simulink model "svpwm3level"  (Simulink 7.1)
settings: Solver=ode3  StartTime=0.0  StopTime=1  RelTol=1e-3
libraries: powerlib x13, simulink x1
(part 2 of 2)

== system svpwm3level/svpwm/Vector status/II/2-1 ==
  m : Inport  OutDataType=sfix(16)  OutScaling=2^0
  Constant1 : Constant  Value=[0 0 0]  OutDataType=sfix(16)  OutScaling=2^0
  Constant11 : Constant  Value=[0 0 0]  OutDataType=sfix(16)  OutScaling=2^0
  Constant12 : Constant  Value=[1 1 0]  OutDataType=sfix(16)  OutScaling=2^0
  Constant13 : Constant  Value=[0 1 0]  OutDataType=sfix(16)  OutScaling=2^0
  Constant2 : Constant  Value=[0 0 -1]  OutDataType=sfix(16)  OutScaling=2^0
  Constant3 : Constant  Value=[0 1 0]  OutDataType=sfix(16)  OutScaling=2^0
  Constant4 : Constant  Value=[1 1 0]  OutDataType=sfix(16)  OutScaling=2^0
  Multiport Switch : MultiPortSwitch  Inputs=7  OutDataType=sfix(16)  OutScaling=2^0  InputSameDT=on
  State : Outport  OutDataType=sfix(16)  OutScaling=2^0
  wires:
  Constant12/1 -> Multiport Switch/2
  Constant13/1 -> Multiport Switch/3
  Constant11/1 -> Multiport Switch/4
  m/1 -> Multiport Switch/1
  Multiport Switch/1 -> State/1
  Constant2/1 -> Multiport Switch/5
  Constant1/1 -> Multiport Switch/6
  Constant3/1 -> Multiport Switch/7
  Constant4/1 -> Multiport Switch/8

== system svpwm3level/svpwm/Vector status/II/2-2 ==
  m : Inport  OutDataType=sfix(16)  OutScaling=2^0
  Constant1 : Constant  Value=[0 0 -1]  OutDataType=sfix(16)  OutScaling=2^0
  Constant2 : Constant  Value=[0 0 0]  OutDataType=sfix(16)  OutScaling=2^0
  Constant3 : Constant  Value=[0 1 0]  OutDataType=sfix(16)  OutScaling=2^0
  Constant6 : Constant  Value=[0 0 -1]  OutDataType=sfix(16)  OutScaling=2^0
  Constant7 : Constant  Value=[0 1 0]  OutDataType=sfix(16)  OutScaling=2^0
  Constant8 : Constant  Value=[0 0 0]  OutDataType=sfix(16)  OutScaling=2^0
  Constant9 : Constant  Value=[-1 0 -1]  OutDataType=sfix(16)  OutScaling=2^0
  Multiport Switch1 : MultiPortSwitch  Inputs=7  OutDataType=sfix(16)  OutScaling=2^0  InputSameDT=on
  State1 : Outport  OutDataType=sfix(16)  OutScaling=2^0
  wires:
  Constant3/1 -> Multiport Switch1/8
  Constant2/1 -> Multiport Switch1/7
  Constant1/1 -> Multiport Switch1/6
  Constant9/1 -> Multiport Switch1/5
  Multiport Switch1/1 -> State1/1
  m/1 -> Multiport Switch1/1
  Constant6/1 -> Multiport Switch1/4
  Constant8/1 -> Multiport Switch1/3
  Constant7/1 -> Multiport Switch1/2

== system svpwm3level/svpwm/Vector status/II/2-3 ==
  m : Inport  OutDataType=sfix(16)  OutScaling=2^0
  Constant1 : Constant  Value=[1 1 0]  OutDataType=sfix(16)  OutScaling=2^0
  Constant11 : Constant  Value=[1 1 0]  OutDataType=sfix(16)  OutScaling=2^0
  Constant12 : Constant  Value=[1 1 -1]  OutDataType=sfix(16)  OutScaling=2^0
  Constant13 : Constant  Value=[0 0 -1]  OutDataType=sfix(16)  OutScaling=2^0
  Constant2 : Constant  Value=[1 1 -1]  OutDataType=sfix(16)  OutScaling=2^0
  Constant3 : Constant  Value=[0 1 -1]  OutDataType=sfix(16)  OutScaling=2^0
  Constant4 : Constant  Value=[0 1 -1]  OutDataType=sfix(16)  OutScaling=2^0
  Multiport Switch2 : MultiPortSwitch  Inputs=7  OutDataType=sfix(16)  OutScaling=2^0  InputSameDT=on
  State2 : Outport  OutDataType=sfix(16)  OutScaling=2^0
  wires:
  Constant1/1 -> Multiport Switch2/8
  Constant2/1 -> Multiport Switch2/7
  Constant3/1 -> Multiport Switch2/6
  Constant13/1 -> Multiport Switch2/5
  Multiport Switch2/1 -> State2/1
  m/1 -> Multiport Switch2/1
  Constant4/1 -> Multiport Switch2/4
  Constant12/1 -> Multiport Switch2/3
  Constant11/1 -> Multiport Switch2/2

== system svpwm3level/svpwm/Vector status/II/2-4 ==
  m : Inport  OutDataType=sfix(16)  OutScaling=2^0
  Constant1 : Constant  Value=[0 1 -1]  OutDataType=sfix(16)  OutScaling=2^0
  Constant14 : Constant  Value=[0 1 -1]  OutDataType=sfix(16)  OutScaling=2^0
  Constant2 : Constant  Value=[0 1 0]  OutDataType=sfix(16)  OutScaling=2^0
  Constant3 : Constant  Value=[1 1 0]  OutDataType=sfix(16)  OutScaling=2^0
  Constant6 : Constant  Value=[1 1 0]  OutDataType=sfix(16)  OutScaling=2^0
  Constant7 : Constant  Value=[0 1 0]  OutDataType=sfix(16)  OutScaling=2^0
  Constant8 : Constant  Value=[0 0 -1]  OutDataType=sfix(16)  OutScaling=2^0
  Multiport Switch1 : MultiPortSwitch  Inputs=7  OutDataType=sfix(16)  OutScaling=2^0  InputSameDT=on
  State : Outport  OutDataType=sfix(16)  OutScaling=2^0
  wires:
  Constant3/1 -> Multiport Switch1/8
  Constant2/1 -> Multiport Switch1/7
  Constant1/1 -> Multiport Switch1/6
  Constant8/1 -> Multiport Switch1/5
  Multiport Switch1/1 -> State/1
  m/1 -> Multiport Switch1/1
  Constant14/1 -> Multiport Switch1/4
  Constant7/1 -> Multiport Switch1/3
  Constant6/1 -> Multiport Switch1/2

== system svpwm3level/svpwm/Vector status/II/2-5 ==
  m : Inport  OutDataType=sfix(16)  OutScaling=2^0
  Constant1 : Constant  Value=[0 0 -1]  OutDataType=sfix(16)  OutScaling=2^0
  Constant16 : Constant  Value=[0 0 -1]  OutDataType=sfix(16)  OutScaling=2^0
  Constant18 : Constant  Value=[0 1 0]  OutDataType=sfix(16)  OutScaling=2^0
  Constant19 : Constant  Value=[0 1 -1]  OutDataType=sfix(16)  OutScaling=2^0
  Constant2 : Constant  Value=[0 1 -1]  OutDataType=sfix(16)  OutScaling=2^0
  Constant20 : Constant  Value=[-1 0 -1]  OutDataType=sfix(16)  OutScaling=2^0
  Constant3 : Constant  Value=[0 1 0]  OutDataType=sfix(16)  OutScaling=2^0
  Multiport Switch3 : MultiPortSwitch  Inputs=7  OutDataType=sfix(16)  OutScaling=2^0  InputSameDT=on
  State : Outport  OutDataType=sfix(16)  OutScaling=2^0
  wires:
  Constant3/1 -> Multiport Switch3/8
  Constant2/1 -> Multiport Switch3/7
  Constant1/1 -> Multiport Switch3/6
  Constant20/1 -> Multiport Switch3/5
  Multiport Switch3/1 -> State/1
  m/1 -> Multiport Switch3/1
  Constant16/1 -> Multiport Switch3/4
  Constant19/1 -> Multiport Switch3/3
  Constant18/1 -> Multiport Switch3/2

== system svpwm3level/svpwm/Vector status/II/2-6 ==
  m : Inport  OutDataType=sfix(16)  OutScaling=2^0
  Constant1 : Constant  Value=[-1 1 -1]  OutDataType=sfix(16)  OutScaling=2^0
  Constant2 : Constant  Value=[0 1 -1]  OutDataType=sfix(16)  OutScaling=2^0
  Constant23 : Constant  Value=[-1 1 -1]  OutDataType=sfix(16)  OutScaling=2^0
  Constant25 : Constant  Value=[0 1 0]  OutDataType=sfix(16)  OutScaling=2^0
  Constant26 : Constant  Value=[0 1 -1]  OutDataType=sfix(16)  OutScaling=2^0
  Constant27 : Constant  Value="[-1 0  -1]"  OutDataType=sfix(16)  OutScaling=2^0
  Constant3 : Constant  Value=[0 1 0]  OutDataType=sfix(16)  OutScaling=2^0
  Multiport Switch4 : MultiPortSwitch  Inputs=7  OutDataType=sfix(16)  OutScaling=2^0  InputSameDT=on
  State : Outport  OutDataType=sfix(16)  OutScaling=2^0
  wires:
  Constant3/1 -> Multiport Switch4/8
  Constant2/1 -> Multiport Switch4/7
  Constant1/1 -> Multiport Switch4/6
  Constant27/1 -> Multiport Switch4/5
  Multiport Switch4/1 -> State/1
  m/1 -> Multiport Switch4/1
  Constant23/1 -> Multiport Switch4/4
  Constant26/1 -> Multiport Switch4/3
  Constant25/1 -> Multiport Switch4/2

== system svpwm3level/svpwm/Vector status/III/3-1 ==
  m : Inport  OutDataType=sfix(16)  OutScaling=2^0
  Constant1 : Constant  Value=[-1 0 0]  OutDataType=sfix(16)  OutScaling=2^0
  Constant11 : Constant  Value=[-1 0 0]  OutDataType=sfix(16)  OutScaling=2^0
  Constant12 : Constant  Value=[0 1 0]  OutDataType=sfix(16)  OutScaling=2^0
  Constant13 : Constant  Value=[0 0 0]  OutDataType=sfix(16)  OutScaling=2^0
  Constant2 : Constant  Value=[-1 0 -1]  OutDataType=sfix(16)  OutScaling=2^0
  Constant3 : Constant  Value=[0 0 0]  OutDataType=sfix(16)  OutScaling=2^0
  Constant4 : Constant  Value=[0 1 0]  OutDataType=sfix(16)  OutScaling=2^0
  Multiport Switch : MultiPortSwitch  Inputs=7  OutDataType=sfix(16)  OutScaling=2^0  InputSameDT=on
  State : Outport  OutDataType=sfix(16)  OutScaling=2^0
  wires:
  Constant12/1 -> Multiport Switch/2
  Constant13/1 -> Multiport Switch/3
  Constant11/1 -> Multiport Switch/4
  m/1 -> Multiport Switch/1
  Multiport Switch/1 -> State/1
  Constant2/1 -> Multiport Switch/5
  Constant1/1 -> Multiport Switch/6
  Constant3/1 -> Multiport Switch/7
  Constant4/1 -> Multiport Switch/8

== system svpwm3level/svpwm/Vector status/III/3-2 ==
  m : Inport  OutDataType=sfix(16)  OutScaling=2^0
  Constant1 : Constant  Value=[0 0 0]  OutDataType=sfix(16)  OutScaling=2^0
  Constant2 : Constant  Value=[0 1 0]  OutDataType=sfix(16)  OutScaling=2^0
  Constant3 : Constant  Value=[0 1 1]  OutDataType=sfix(16)  OutScaling=2^0
  Constant6 : Constant  Value=[0 0 0]  OutDataType=sfix(16)  OutScaling=2^0
  Constant7 : Constant  Value=[0 1 1]  OutDataType=sfix(16)  OutScaling=2^0
  Constant8 : Constant  Value=[0 1 0]  OutDataType=sfix(16)  OutScaling=2^0
  Constant9 : Constant  Value=[-1 0 0]  OutDataType=sfix(16)  OutScaling=2^0
  Multiport Switch1 : MultiPortSwitch  Inputs=7  OutDataType=sfix(16)  OutScaling=2^0  InputSameDT=on
  State : Outport  OutDataType=sfix(16)  OutScaling=2^0
  wires:
  Constant3/1 -> Multiport Switch1/8
  Constant2/1 -> Multiport Switch1/7
  Constant1/1 -> Multiport Switch1/6
  Constant9/1 -> Multiport Switch1/5
  Multiport Switch1/1 -> State/1
  m/1 -> Multiport Switch1/1
  Constant6/1 -> Multiport Switch1/4
  Constant8/1 -> Multiport Switch1/3
  Constant7/1 -> Multiport Switch1/2

== system svpwm3level/svpwm/Vector status/III/3-3 ==
  m : Inport  OutDataType=sfix(16)  OutScaling=2^0
  Constant1 : Constant  Value=[-1 1 -1]  OutDataType=sfix(16)  OutScaling=2^0
  Constant11 : Constant  Value=[0 1 0]  OutDataType=sfix(16)  OutScaling=2^0
  Constant12 : Constant  Value=[-1 1 0]  OutDataType=sfix(16)  OutScaling=2^0
  Constant13 : Constant  Value=[-1 0 -1]  OutDataType=sfix(16)  OutScaling=2^0
  Constant2 : Constant  Value=[-1 1 0]  OutDataType=sfix(16)  OutScaling=2^0
  Constant3 : Constant  Value=[0 1 0]  OutDataType=sfix(16)  OutScaling=2^0
  Constant4 : Constant  Value=[-1 1 -1]  OutDataType=sfix(16)  OutScaling=2^0
  Multiport Switch2 : MultiPortSwitch  Inputs=7  OutDataType=sfix(16)  OutScaling=2^0  InputSameDT=on
  State2 : Outport  OutDataType=sfix(16)  OutScaling=2^0
  wires:
  Constant3/1 -> Multiport Switch2/8
  Constant2/1 -> Multiport Switch2/7
  Constant1/1 -> Multiport Switch2/6
  Constant13/1 -> Multiport Switch2/5
  Multiport Switch2/1 -> State2/1
  m/1 -> Multiport Switch2/1
  Constant4/1 -> Multiport Switch2/4
  Constant12/1 -> Multiport Switch2/3
  Constant11/1 -> Multiport Switch2/2

== system svpwm3level/svpwm/Vector status/III/3-4 ==
  m : Inport  OutDataType=sfix(16)  OutScaling=2^0
  Constant1 : Constant  Value=[-1 0 0]  OutDataType=sfix(16)  OutScaling=2^0
  Constant14 : Constant  Value=[-1 0 0]  OutDataType=sfix(16)  OutScaling=2^0
  Constant2 : Constant  Value=[-1 1 0]  OutDataType=sfix(16)  OutScaling=2^0
  Constant3 : Constant  Value=[0 1 0]  OutDataType=sfix(16)  OutScaling=2^0
  Constant6 : Constant  Value=[0 1 0]  OutDataType=sfix(16)  OutScaling=2^0
  Constant7 : Constant  Value=[-1 1 0]  OutDataType=sfix(16)  OutScaling=2^0
  Constant8 : Constant  Value=[-1 0 -1]  OutDataType=sfix(16)  OutScaling=2^0
  Multiport Switch1 : MultiPortSwitch  Inputs=7  OutDataType=sfix(16)  OutScaling=2^0  InputSameDT=on
  State : Outport  OutDataType=sfix(16)  OutScaling=2^0
  wires:
  Constant3/1 -> Multiport Switch1/8
  Constant2/1 -> Multiport Switch1/7
  Constant1/1 -> Multiport Switch1/6
  Constant8/1 -> Multiport Switch1/5
  Multiport Switch1/1 -> State/1
  m/1 -> Multiport Switch1/1
  Constant14/1 -> Multiport Switch1/4
  Constant7/1 -> Multiport Switch1/3
  Constant6/1 -> Multiport Switch1/2

== system svpwm3level/svpwm/Vector status/III/3-5 ==
  m : Inport  OutDataType=sfix(16)  OutScaling=2^0
  Constant1 : Constant  Value=[-1 1 0]  OutDataType=sfix(16)  OutScaling=2^0
  Constant16 : Constant  Value=[-1 1 0]  OutDataType=sfix(16)  OutScaling=2^0
  Constant18 : Constant  Value=[0 1 1]  OutDataType=sfix(16)  OutScaling=2^0
  Constant19 : Constant  Value=[0 1 0]  OutDataType=sfix(16)  OutScaling=2^0
  Constant2 : Constant  Value=[0 1 0]  OutDataType=sfix(16)  OutScaling=2^0
  Constant20 : Constant  Value=[-1 0 0]  OutDataType=sfix(16)  OutScaling=2^0
  Constant3 : Constant  Value=[0 1 1]  OutDataType=sfix(16)  OutScaling=2^0
  Multiport Switch3 : MultiPortSwitch  Inputs=7  OutDataType=sfix(16)  OutScaling=2^0  InputSameDT=on
  State : Outport  OutDataType=sfix(16)  OutScaling=2^0
  wires:
  Constant3/1 -> Multiport Switch3/8
  Constant2/1 -> Multiport Switch3/7
  Constant1/1 -> Multiport Switch3/6
  Constant20/1 -> Multiport Switch3/5
  Multiport Switch3/1 -> State/1
  m/1 -> Multiport Switch3/1
  Constant16/1 -> Multiport Switch3/4
  Constant19/1 -> Multiport Switch3/3
  Constant18/1 -> Multiport Switch3/2

== system svpwm3level/svpwm/Vector status/III/3-6 ==
  m : Inport  OutDataType=sfix(16)  OutScaling=2^0
  Constant1 : Constant  Value=[-1 1 0]  OutDataType=sfix(16)  OutScaling=2^0
  Constant2 : Constant  Value=[-1 1 1]  OutDataType=sfix(16)  OutScaling=2^0
  Constant23 : Constant  Value=[-1 1 0]  OutDataType=sfix(16)  OutScaling=2^0
  Constant25 : Constant  Value=[0 1 1]  OutDataType=sfix(16)  OutScaling=2^0
  Constant26 : Constant  Value=[-1 1 1]  OutDataType=sfix(16)  OutScaling=2^0
  Constant27 : Constant  Value=[-1 0 0]  OutDataType=sfix(16)  OutScaling=2^0
  Constant3 : Constant  Value=[0 1 1]  OutDataType=sfix(16)  OutScaling=2^0
  Multiport Switch4 : MultiPortSwitch  Inputs=7  OutDataType=sfix(16)  OutScaling=2^0  InputSameDT=on
  State : Outport  OutDataType=sfix(16)  OutScaling=2^0
  wires:
  Constant3/1 -> Multiport Switch4/8
  Constant2/1 -> Multiport Switch4/7
  Constant1/1 -> Multiport Switch4/6
  Constant27/1 -> Multiport Switch4/5
  Multiport Switch4/1 -> State/1
  m/1 -> Multiport Switch4/1
  Constant23/1 -> Multiport Switch4/4
  Constant26/1 -> Multiport Switch4/3
  Constant25/1 -> Multiport Switch4/2

== system svpwm3level/svpwm/Vector status/IV/4-1 ==
  m : Inport  OutDataType=sfix(16)  OutScaling=2^0
  Constant1 : Constant  Value=[0 0 0]  OutDataType=sfix(16)  OutScaling=2^0
  Constant11 : Constant  Value=[0 0 0]  OutDataType=sfix(16)  OutScaling=2^0
  Constant12 : Constant  Value=[0 1 1]  OutDataType=sfix(16)  OutScaling=2^0
  Constant13 : Constant  Value=[0 0 1]  OutDataType=sfix(16)  OutScaling=2^0
  Constant2 : Constant  Value=[-1 0 0]  OutDataType=sfix(16)  OutScaling=2^0
  Constant3 : Constant  Value=[0 0 1]  OutDataType=sfix(16)  OutScaling=2^0
  Constant4 : Constant  Value=[0 1 1]  OutDataType=sfix(16)  OutScaling=2^0
  Multiport Switch : MultiPortSwitch  Inputs=7  OutDataType=sfix(16)  OutScaling=2^0  InputSameDT=on
  State : Outport  OutDataType=sfix(16)  OutScaling=2^0
  wires:
  Constant12/1 -> Multiport Switch/2
  Constant13/1 -> Multiport Switch/3
  Constant11/1 -> Multiport Switch/4
  m/1 -> Multiport Switch/1
  Multiport Switch/1 -> State/1
  Constant2/1 -> Multiport Switch/5
  Constant1/1 -> Multiport Switch/6
  Constant3/1 -> Multiport Switch/7
  Constant4/1 -> Multiport Switch/8

== system svpwm3level/svpwm/Vector status/IV/4-2 ==
  m : Inport  OutDataType=sfix(16)  OutScaling=2^0
  Constant1 : Constant  Value=[-1 0 0]  OutDataType=sfix(16)  OutScaling=2^0
  Constant2 : Constant  Value=[0 0 0]  OutDataType=sfix(16)  OutScaling=2^0
  Constant3 : Constant  Value=[0 0 1]  OutDataType=sfix(16)  OutScaling=2^0
  Constant6 : Constant  Value=[-1 0 0]  OutDataType=sfix(16)  OutScaling=2^0
  Constant7 : Constant  Value=[0 0 1]  OutDataType=sfix(16)  OutScaling=2^0
  Constant8 : Constant  Value=[0 0 0]  OutDataType=sfix(16)  OutScaling=2^0
  Constant9 : Constant  Value=[-1 -1 0]  OutDataType=sfix(16)  OutScaling=2^0
  Multiport Switch1 : MultiPortSwitch  Inputs=7  OutDataType=sfix(16)  OutScaling=2^0  InputSameDT=on
  State : Outport  OutDataType=sfix(16)  OutScaling=2^0
  wires:
  Constant3/1 -> Multiport Switch1/8
  Constant2/1 -> Multiport Switch1/7
  Constant1/1 -> Multiport Switch1/6
  Constant9/1 -> Multiport Switch1/5
  Multiport Switch1/1 -> State/1
  m/1 -> Multiport Switch1/1
  Constant6/1 -> Multiport Switch1/4
  Constant8/1 -> Multiport Switch1/3
  Constant7/1 -> Multiport Switch1/2

== system svpwm3level/svpwm/Vector status/IV/4-3 ==
  m : Inport  OutDataType=sfix(16)  OutScaling=2^0
  Constant1 : Constant  Value=[-1 0 1]  OutDataType=sfix(16)  OutScaling=2^0
  Constant11 : Constant  Value="[0 1  1]"  OutDataType=sfix(16)  OutScaling=2^0
  Constant12 : Constant  Value=[-1 1 1]  OutDataType=sfix(16)  OutScaling=2^0
  Constant13 : Constant  Value=[-1 0 0]  OutDataType=sfix(16)  OutScaling=2^0
  Constant2 : Constant  Value=[-1 1 1]  OutDataType=sfix(16)  OutScaling=2^0
  Constant3 : Constant  Value="[0 1  1]"  OutDataType=sfix(16)  OutScaling=2^0
  Constant4 : Constant  Value=[-1 0 1]  OutDataType=sfix(16)  OutScaling=2^0
  Multiport Switch2 : MultiPortSwitch  Inputs=7  OutDataType=sfix(16)  OutScaling=2^0  InputSameDT=on
  State2 : Outport  OutDataType=sfix(16)  OutScaling=2^0
  wires:
  Constant3/1 -> Multiport Switch2/8
  Constant2/1 -> Multiport Switch2/7
  Constant1/1 -> Multiport Switch2/6
  Constant13/1 -> Multiport Switch2/5
  Multiport Switch2/1 -> State2/1
  m/1 -> Multiport Switch2/1
  Constant4/1 -> Multiport Switch2/4
  Constant12/1 -> Multiport Switch2/3
  Constant11/1 -> Multiport Switch2/2

== system svpwm3level/svpwm/Vector status/IV/4-4 ==
  m : Inport  OutDataType=sfix(16)  OutScaling=2^0
  Constant1 : Constant  Value=[-1 0 1]  OutDataType=sfix(16)  OutScaling=2^0
  Constant14 : Constant  Value=[-1 0 1]  OutDataType=sfix(16)  OutScaling=2^0
  Constant2 : Constant  Value=[0 0 1]  OutDataType=sfix(16)  OutScaling=2^0
  Constant3 : Constant  Value=[0 1 1]  OutDataType=sfix(16)  OutScaling=2^0
  Constant6 : Constant  Value=[0 1 1]  OutDataType=sfix(16)  OutScaling=2^0
  Constant7 : Constant  Value=[0 0 1]  OutDataType=sfix(16)  OutScaling=2^0
  Constant8 : Constant  Value=[-1 0 0]  OutDataType=sfix(16)  OutScaling=2^0
  Multiport Switch1 : MultiPortSwitch  Inputs=7  OutDataType=sfix(16)  OutScaling=2^0  InputSameDT=on
  State : Outport  OutDataType=sfix(16)  OutScaling=2^0
  wires:
  Constant3/1 -> Multiport Switch1/8
  Constant2/1 -> Multiport Switch1/7
  Constant1/1 -> Multiport Switch1/6
  Constant8/1 -> Multiport Switch1/5
  Multiport Switch1/1 -> State/1
  m/1 -> Multiport Switch1/1
  Constant14/1 -> Multiport Switch1/4
  Constant7/1 -> Multiport Switch1/3
  Constant6/1 -> Multiport Switch1/2

== system svpwm3level/svpwm/Vector status/IV/4-5 ==
  m : Inport  OutDataType=sfix(16)  OutScaling=2^0
  Constant1 : Constant  Value=[0 0 1]  OutDataType=sfix(16)  OutScaling=2^0
  Constant16 : Constant  Value=[-1 0 0]  OutDataType=sfix(16)  OutScaling=2^0
  Constant18 : Constant  Value=[0 0 1]  OutDataType=sfix(16)  OutScaling=2^0
  Constant19 : Constant  Value=[-1 0 1]  OutDataType=sfix(16)  OutScaling=2^0
  Constant2 : Constant  Value=[-1 0 1]  OutDataType=sfix(16)  OutScaling=2^0
  Constant20 : Constant  Value=[-1 -1 0]  OutDataType=sfix(16)  OutScaling=2^0
  Constant3 : Constant  Value=[-1 0 0]  OutDataType=sfix(16)  OutScaling=2^0
  Multiport Switch3 : MultiPortSwitch  Inputs=7  OutDataType=sfix(16)  OutScaling=2^0  InputSameDT=on
  State4 : Outport  OutDataType=sfix(16)  OutScaling=2^0
  wires:
  Constant1/1 -> Multiport Switch3/8
  Constant2/1 -> Multiport Switch3/7
  Constant3/1 -> Multiport Switch3/6
  Constant20/1 -> Multiport Switch3/5
  Multiport Switch3/1 -> State4/1
  m/1 -> Multiport Switch3/1
  Constant16/1 -> Multiport Switch3/4
  Constant19/1 -> Multiport Switch3/3
  Constant18/1 -> Multiport Switch3/2

== system svpwm3level/svpwm/Vector status/IV/4-6 ==
  m : Inport  OutDataType=sfix(16)  OutScaling=2^0
  Constant1 : Constant  Value=[-1 -1 1]  OutDataType=sfix(16)  OutScaling=2^0
  Constant2 : Constant  Value=[-1 0 1]  OutDataType=sfix(16)  OutScaling=2^0
  Constant23 : Constant  Value=[-1 -1 1]  OutDataType=sfix(16)  OutScaling=2^0
  Constant25 : Constant  Value=[0 0 1]  OutDataType=sfix(16)  OutScaling=2^0
  Constant26 : Constant  Value=[-1 0 1]  OutDataType=sfix(16)  OutScaling=2^0
  Constant27 : Constant  Value=[-1 -1 0]  OutDataType=sfix(16)  OutScaling=2^0
  Constant3 : Constant  Value=[0 0 1]  OutDataType=sfix(16)  OutScaling=2^0
  Multiport Switch4 : MultiPortSwitch  Inputs=7  OutDataType=sfix(16)  OutScaling=2^0  InputSameDT=on
  State : Outport  OutDataType=sfix(16)  OutScaling=2^0
  wires:
  Constant3/1 -> Multiport Switch4/8
  Constant2/1 -> Multiport Switch4/7
  Constant1/1 -> Multiport Switch4/6
  Constant27/1 -> Multiport Switch4/5
  Multiport Switch4/1 -> State/1
  m/1 -> Multiport Switch4/1
  Constant23/1 -> Multiport Switch4/4
  Constant26/1 -> Multiport Switch4/3
  Constant25/1 -> Multiport Switch4/2

== system svpwm3level/svpwm/Vector status/V/5-1 ==
  m : Inport  OutDataType=sfix(16)  OutScaling=2^0
  Constant1 : Constant  Value=[0 -1 0]  OutDataType=sfix(16)  OutScaling=2^0
  Constant11 : Constant  Value=[0 -1 0]  OutDataType=sfix(16)  OutScaling=2^0
  Constant12 : Constant  Value=[0 0 1]  OutDataType=sfix(16)  OutScaling=2^0
  Constant13 : Constant  Value=[0 0 0]  OutDataType=sfix(16)  OutScaling=2^0
  Constant2 : Constant  Value=[-1 -1 0]  OutDataType=sfix(16)  OutScaling=2^0
  Constant3 : Constant  Value=[0 0 0]  OutDataType=sfix(16)  OutScaling=2^0
  Constant4 : Constant  Value=[0 0 1]  OutDataType=sfix(16)  OutScaling=2^0
  Multiport Switch : MultiPortSwitch  Inputs=7  OutDataType=sfix(16)  OutScaling=2^0  InputSameDT=on
  State : Outport  OutDataType=sfix(16)  OutScaling=2^0
  wires:
  Constant12/1 -> Multiport Switch/2
  Constant13/1 -> Multiport Switch/3
  Constant11/1 -> Multiport Switch/4
  m/1 -> Multiport Switch/1
  Multiport Switch/1 -> State/1
  Constant2/1 -> Multiport Switch/5
  Constant1/1 -> Multiport Switch/6
  Constant3/1 -> Multiport Switch/7
  Constant4/1 -> Multiport Switch/8

== system svpwm3level/svpwm/Vector status/V/5-2 ==
  m : Inport  OutDataType=sfix(16)  OutScaling=2^0
  Constant1 : Constant  Value=[0 0 0]  OutDataType=sfix(16)  OutScaling=2^0
  Constant2 : Constant  Value=[0 0 1]  OutDataType=sfix(16)  OutScaling=2^0
  Constant3 : Constant  Value=[1 0 1]  OutDataType=sfix(16)  OutScaling=2^0
  Constant6 : Constant  Value=[0 0 0]  OutDataType=sfix(16)  OutScaling=2^0
  Constant7 : Constant  Value=[1 0 1]  OutDataType=sfix(16)  OutScaling=2^0
  Constant8 : Constant  Value=[0 0 1]  OutDataType=sfix(16)  OutScaling=2^0
  Constant9 : Constant  Value=[0 -1 0]  OutDataType=sfix(16)  OutScaling=2^0
  Multiport Switch1 : MultiPortSwitch  Inputs=7  OutDataType=sfix(16)  OutScaling=2^0  InputSameDT=on
  State1 : Outport  OutDataType=sfix(16)  OutScaling=2^0
  wires:
  Constant3/1 -> Multiport Switch1/8
  Constant2/1 -> Multiport Switch1/7
  Constant1/1 -> Multiport Switch1/6
  Constant9/1 -> Multiport Switch1/5
  Multiport Switch1/1 -> State1/1
  m/1 -> Multiport Switch1/1
  Constant6/1 -> Multiport Switch1/4
  Constant8/1 -> Multiport Switch1/3
  Constant7/1 -> Multiport Switch1/2

== system svpwm3level/svpwm/Vector status/V/5-3 ==
  m : Inport  OutDataType=sfix(16)  OutScaling=2^0
  Constant1 : Constant  Value=[0 0 1]  OutDataType=sfix(16)  OutScaling=2^0
  Constant11 : Constant  Value=[0 0 1]  OutDataType=sfix(16)  OutScaling=2^0
  Constant12 : Constant  Value=[0 -1 1]  OutDataType=sfix(16)  OutScaling=2^0
  Constant13 : Constant  Value=[-1 -1 0]  OutDataType=sfix(16)  OutScaling=2^0
  Constant2 : Constant  Value=[0 -1 1]  OutDataType=sfix(16)  OutScaling=2^0
  Constant3 : Constant  Value=[-1 -1 1]  OutDataType=sfix(16)  OutScaling=2^0
  Constant4 : Constant  Value=[-1 -1 1]  OutDataType=sfix(16)  OutScaling=2^0
  Multiport Switch2 : MultiPortSwitch  Inputs=7  OutDataType=sfix(16)  OutScaling=2^0  InputSameDT=on
  State2 : Outport  OutDataType=sfix(16)  OutScaling=2^0
  wires:
  Constant1/1 -> Multiport Switch2/8
  Constant2/1 -> Multiport Switch2/7
  Constant3/1 -> Multiport Switch2/6
  Constant13/1 -> Multiport Switch2/5
  Multiport Switch2/1 -> State2/1
  m/1 -> Multiport Switch2/1
  Constant4/1 -> Multiport Switch2/4
  Constant12/1 -> Multiport Switch2/3
  Constant11/1 -> Multiport Switch2/2

== system svpwm3level/svpwm/Vector status/V/5-4 ==
  m : Inport  OutDataType=sfix(16)  OutScaling=2^0
  Constant1 : Constant  Value=[0 -1 0]  OutDataType=sfix(16)  OutScaling=2^0
  Constant14 : Constant  Value=[0 -1 0]  OutDataType=sfix(16)  OutScaling=2^0
  Constant2 : Constant  Value=[0 -1 1]  OutDataType=sfix(16)  OutScaling=2^0
  Constant3 : Constant  Value=[0 0 1]  OutDataType=sfix(16)  OutScaling=2^0
  Constant6 : Constant  Value=[0 0 1]  OutDataType=sfix(16)  OutScaling=2^0
  Constant7 : Constant  Value=[0 -1 1]  OutDataType=sfix(16)  OutScaling=2^0
  Constant8 : Constant  Value=[-1 -1 0]  OutDataType=sfix(16)  OutScaling=2^0
  Multiport Switch1 : MultiPortSwitch  Inputs=7  OutDataType=sfix(16)  OutScaling=2^0  InputSameDT=on
  State3 : Outport  OutDataType=sfix(16)  OutScaling=2^0
  wires:
  Constant3/1 -> Multiport Switch1/8
  Constant2/1 -> Multiport Switch1/7
  Constant1/1 -> Multiport Switch1/6
  Constant8/1 -> Multiport Switch1/5
  Multiport Switch1/1 -> State3/1
  m/1 -> Multiport Switch1/1
  Constant14/1 -> Multiport Switch1/4
  Constant7/1 -> Multiport Switch1/3
  Constant6/1 -> Multiport Switch1/2

== system svpwm3level/svpwm/Vector status/V/5-5 ==
  m : Inport  OutDataType=sfix(16)  OutScaling=2^0
  Constant1 : Constant  Value=[0 -1 1]  OutDataType=sfix(16)  OutScaling=2^0
  Constant16 : Constant  Value=[0 -1 1]  OutDataType=sfix(16)  OutScaling=2^0
  Constant18 : Constant  Value=[1 0 1]  OutDataType=sfix(16)  OutScaling=2^0
  Constant19 : Constant  Value=[0 0 1]  OutDataType=sfix(16)  OutScaling=2^0
  Constant2 : Constant  Value=[0 0 1]  OutDataType=sfix(16)  OutScaling=2^0
  Constant20 : Constant  Value=[0 -1 0]  OutDataType=sfix(16)  OutScaling=2^0
  Constant3 : Constant  Value=[1 0 1]  OutDataType=sfix(16)  OutScaling=2^0
  Multiport Switch3 : MultiPortSwitch  Inputs=7  OutDataType=sfix(16)  OutScaling=2^0  InputSameDT=on
  State4 : Outport  OutDataType=sfix(16)  OutScaling=2^0
  wires:
  Constant3/1 -> Multiport Switch3/8
  Constant2/1 -> Multiport Switch3/7
  Constant1/1 -> Multiport Switch3/6
  Constant20/1 -> Multiport Switch3/5
  Multiport Switch3/1 -> State4/1
  m/1 -> Multiport Switch3/1
  Constant16/1 -> Multiport Switch3/4
  Constant19/1 -> Multiport Switch3/3
  Constant18/1 -> Multiport Switch3/2

== system svpwm3level/svpwm/Vector status/V/5-6 ==
  m : Inport  OutDataType=sfix(16)  OutScaling=2^0
  Constant1 : Constant  Value=[1 0 1]  OutDataType=sfix(16)  OutScaling=2^0
  Constant2 : Constant  Value=[1 -1 1]  OutDataType=sfix(16)  OutScaling=2^0
  Constant23 : Constant  Value=[0 -1 1]  OutDataType=sfix(16)  OutScaling=2^0
  Constant25 : Constant  Value=[1 0 1]  OutDataType=sfix(16)  OutScaling=2^0
  Constant26 : Constant  Value=[1 -1 1]  OutDataType=sfix(16)  OutScaling=2^0
  Constant27 : Constant  Value=[0 -1 0]  OutDataType=sfix(16)  OutScaling=2^0
  Constant3 : Constant  Value=[0 -1 1]  OutDataType=sfix(16)  OutScaling=2^0
  Multiport Switch4 : MultiPortSwitch  Inputs=7  OutDataType=sfix(16)  OutScaling=2^0  InputSameDT=on
  State : Outport  OutDataType=sfix(16)  OutScaling=2^0
  wires:
  Constant1/1 -> Multiport Switch4/8
  Constant2/1 -> Multiport Switch4/7
  Constant3/1 -> Multiport Switch4/6
  Constant27/1 -> Multiport Switch4/5
  Multiport Switch4/1 -> State/1
  m/1 -> Multiport Switch4/1
  Constant23/1 -> Multiport Switch4/4
  Constant26/1 -> Multiport Switch4/3
  Constant25/1 -> Multiport Switch4/2

== system svpwm3level/svpwm/Vector status/VI/6-1 ==
  m : Inport  OutDataType=sfix(16)  OutScaling=2^0
  Constant1 : Constant  Value=[1 0 0]  OutDataType=sfix(16)  OutScaling=2^0
  Constant11 : Constant  Value=[0 0 0]  OutDataType=sfix(16)  OutScaling=2^0
  Constant12 : Constant  Value=[1 0 1]  OutDataType=sfix(16)  OutScaling=2^0
  Constant13 : Constant  Value=[1 0 0]  OutDataType=sfix(16)  OutScaling=2^0
  Constant2 : Constant  Value=[0 -1 0]  OutDataType=sfix(16)  OutScaling=2^0
  Constant3 : Constant  Value=[0 0 0]  OutDataType=sfix(16)  OutScaling=2^0
  Constant4 : Constant  Value=[1 0 1]  OutDataType=sfix(16)  OutScaling=2^0
  Multiport Switch : MultiPortSwitch  Inputs=7  OutDataType=sfix(16)  OutScaling=2^0  InputSameDT=on
  State : Outport  OutDataType=sfix(16)  OutScaling=2^0
  wires:
  Constant12/1 -> Multiport Switch/2
  Constant13/1 -> Multiport Switch/3
  Constant11/1 -> Multiport Switch/4
  m/1 -> Multiport Switch/1
  Multiport Switch/1 -> State/1
  Constant2/1 -> Multiport Switch/5
  Constant3/1 -> Multiport Switch/6
  Constant1/1 -> Multiport Switch/7
  Constant4/1 -> Multiport Switch/8

== system svpwm3level/svpwm/Vector status/VI/6-2 ==
  m : Inport  OutDataType=sfix(16)  OutScaling=2^0
  Constant1 : Constant  Value=[0 -1 0]  OutDataType=sfix(16)  OutScaling=2^0
  Constant2 : Constant  Value=[0 0 0]  OutDataType=sfix(16)  OutScaling=2^0
  Constant3 : Constant  Value=[1 0 0]  OutDataType=sfix(16)  OutScaling=2^0
  Constant6 : Constant  Value=[0 -1 0]  OutDataType=sfix(16)  OutScaling=2^0
  Constant7 : Constant  Value=[1 0 0]  OutDataType=sfix(16)  OutScaling=2^0
  Constant8 : Constant  Value=[0 0 0]  OutDataType=sfix(16)  OutScaling=2^0
  Constant9 : Constant  Value=[0 -1 -1]  OutDataType=sfix(16)  OutScaling=2^0
  Multiport Switch1 : MultiPortSwitch  Inputs=7  OutDataType=sfix(16)  OutScaling=2^0  InputSameDT=on
  State : Outport  OutDataType=sfix(16)  OutScaling=2^0
  wires:
  Constant3/1 -> Multiport Switch1/8
  Constant2/1 -> Multiport Switch1/7
  Constant1/1 -> Multiport Switch1/6
  Constant9/1 -> Multiport Switch1/5
  Multiport Switch1/1 -> State/1
  m/1 -> Multiport Switch1/1
  Constant6/1 -> Multiport Switch1/4
  Constant8/1 -> Multiport Switch1/3
  Constant7/1 -> Multiport Switch1/2

== system svpwm3level/svpwm/Vector status/VI/6-3 ==
  m : Inport  OutDataType=sfix(16)  OutScaling=2^0
  Constant1 : Constant  Value=[1 -1 0]  OutDataType=sfix(16)  OutScaling=2^0
  Constant11 : Constant  Value=[1 0 1]  OutDataType=sfix(16)  OutScaling=2^0
  Constant12 : Constant  Value=[1 -1 1]  OutDataType=sfix(16)  OutScaling=2^0
  Constant13 : Constant  Value=[0 -1 0]  OutDataType=sfix(16)  OutScaling=2^0
  Constant2 : Constant  Value=[1 -1 1]  OutDataType=sfix(16)  OutScaling=2^0
  Constant3 : Constant  Value=[1 0 1]  OutDataType=sfix(16)  OutScaling=2^0
  Constant4 : Constant  Value=[1 -1 0]  OutDataType=sfix(16)  OutScaling=2^0
  Multiport Switch2 : MultiPortSwitch  Inputs=7  OutDataType=sfix(16)  OutScaling=2^0  InputSameDT=on
  State2 : Outport  OutDataType=sfix(16)  OutScaling=2^0
  wires:
  Constant3/1 -> Multiport Switch2/8
  Constant2/1 -> Multiport Switch2/7
  Constant1/1 -> Multiport Switch2/6
  Constant13/1 -> Multiport Switch2/5
  Multiport Switch2/1 -> State2/1
  m/1 -> Multiport Switch2/1
  Constant4/1 -> Multiport Switch2/4
  Constant12/1 -> Multiport Switch2/3
  Constant11/1 -> Multiport Switch2/2

== system svpwm3level/svpwm/Vector status/VI/6-4 ==
  m : Inport  OutDataType=sfix(16)  OutScaling=2^0
  Constant1 : Constant  Value=[1 0 1]  OutDataType=sfix(16)  OutScaling=2^0
  Constant14 : Constant  Value="[1 -1  0]"  OutDataType=sfix(16)  OutScaling=2^0
  Constant2 : Constant  Value=[1 0 0]  OutDataType=sfix(16)  OutScaling=2^0
  Constant3 : Constant  Value="[1 -1  0]"  OutDataType=sfix(16)  OutScaling=2^0
  Constant6 : Constant  Value=[1 0 1]  OutDataType=sfix(16)  OutScaling=2^0
  Constant7 : Constant  Value=[1 0 0]  OutDataType=sfix(16)  OutScaling=2^0
  Constant8 : Constant  Value="[0 -1  0]"  OutDataType=sfix(16)  OutScaling=2^0
  Multiport Switch1 : MultiPortSwitch  Inputs=7  OutDataType=sfix(16)  OutScaling=2^0  InputSameDT=on
  State3 : Outport  OutDataType=sfix(16)  OutScaling=2^0
  wires:
  Constant1/1 -> Multiport Switch1/8
  Constant2/1 -> Multiport Switch1/7
  Constant3/1 -> Multiport Switch1/6
  Constant8/1 -> Multiport Switch1/5
  Multiport Switch1/1 -> State3/1
  m/1 -> Multiport Switch1/1
  Constant14/1 -> Multiport Switch1/4
  Constant7/1 -> Multiport Switch1/3
  Constant6/1 -> Multiport Switch1/2

== system svpwm3level/svpwm/Vector status/VI/6-5 ==
  m : Inport  OutDataType=sfix(16)  OutScaling=2^0
  Constant1 : Constant  Value=[0 -1 0]  OutDataType=sfix(16)  OutScaling=2^0
  Constant16 : Constant  Value=[0 -1 0]  OutDataType=sfix(16)  OutScaling=2^0
  Constant18 : Constant  Value=[1 0 0]  OutDataType=sfix(16)  OutScaling=2^0
  Constant19 : Constant  Value=[1 -1 0]  OutDataType=sfix(16)  OutScaling=2^0
  Constant2 : Constant  Value=[1 -1 0]  OutDataType=sfix(16)  OutScaling=2^0
  Constant20 : Constant  Value=[0 -1 -1]  OutDataType=sfix(16)  OutScaling=2^0
  Constant3 : Constant  Value=[1 0 0]  OutDataType=sfix(16)  OutScaling=2^0
  Multiport Switch3 : MultiPortSwitch  Inputs=7  OutDataType=sfix(16)  OutScaling=2^0  InputSameDT=on
  State4 : Outport  OutDataType=sfix(16)  OutScaling=2^0
  wires:
  Constant3/1 -> Multiport Switch3/8
  Constant2/1 -> Multiport Switch3/7
  Constant1/1 -> Multiport Switch3/6
  Constant20/1 -> Multiport Switch3/5
  Multiport Switch3/1 -> State4/1
  m/1 -> Multiport Switch3/1
  Constant16/1 -> Multiport Switch3/4
  Constant19/1 -> Multiport Switch3/3
  Constant18/1 -> Multiport Switch3/2

== system svpwm3level/svpwm/Vector status/VI/6-6 ==
  m : Inport  OutDataType=sfix(16)  OutScaling=2^0
  Constant1 : Constant  Value=[1 -1 -1]  OutDataType=sfix(16)  OutScaling=2^0
  Constant2 : Constant  Value=[1 -1 0]  OutDataType=sfix(16)  OutScaling=2^0
  Constant23 : Constant  Value=[1 -1 -1]  OutDataType=sfix(16)  OutScaling=2^0
  Constant25 : Constant  Value=[1 0 0]  OutDataType=sfix(16)  OutScaling=2^0
  Constant26 : Constant  Value=[1 -1 0]  OutDataType=sfix(16)  OutScaling=2^0
  Constant27 : Constant  Value=[0 -1 -1]  OutDataType=sfix(16)  OutScaling=2^0
  Constant3 : Constant  Value=[1 0 0]  OutDataType=sfix(16)  OutScaling=2^0
  Multiport Switch4 : MultiPortSwitch  Inputs=7  OutDataType=sfix(16)  OutScaling=2^0  InputSameDT=on
  State : Outport  OutDataType=sfix(16)  OutScaling=2^0
  wires:
  Constant3/1 -> Multiport Switch4/8
  Constant2/1 -> Multiport Switch4/7
  Constant1/1 -> Multiport Switch4/6
  Constant27/1 -> Multiport Switch4/5
  Multiport Switch4/1 -> State/1
  m/1 -> Multiport Switch4/1
  Constant23/1 -> Multiport Switch4/4
  Constant26/1 -> Multiport Switch4/3
  Constant25/1 -> Multiport Switch4/2
